simulink model "g"  (Simulink 7.9)
settings: Solver=ode45  StartTime=0.0  StopTime=10.0  RelTol=1e-3
libraries: dspsigops x2
settings Model: Creator=Mihail  LastModifiedBy=Mihail
settings ConfigurationSet: Description=SimMechanics 2G

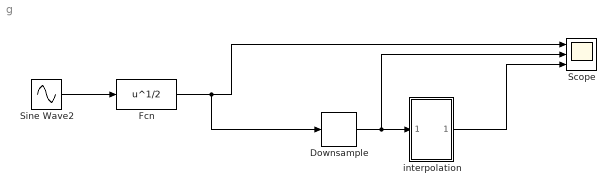
== system g ==
  Downsample : dspsigops/Downsample  N=4  phase=0  RateOptions=Enforce single-rate processing  smode=Allow multirate  fmode=Maintain input frame size  ic=0
  Fcn : Fcn  Expr=u^1/2
  Scope : Scope  NumInputPorts=3
      settings: YMin=-5~-5~-5  YMax=5~5~5
  Sine Wave2 : Sin  Amplitude=1000  Frequency=4  Phase=2*pi  SampleTime=0.01  VectorParams1D=off
  interpolation : Subsystem
  wires:
  Downsample/1 -> interpolation/1(In1), Scope/2
  interpolation/1(Out1) -> Scope/3
  Sine Wave2/1 -> Fcn/1
  Fcn/1 -> Scope/1, Downsample/1

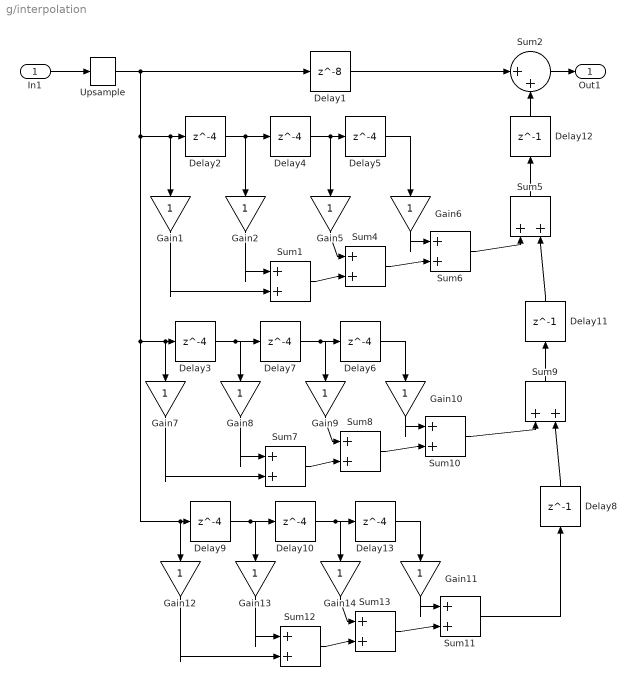
== system g/interpolation ==
  In1 : Inport
  Delay1 : Delay  DelayLength=8
  Delay{2..7,9..10,13} (9 alike) : Delay  DelayLength=4
  Delay11 : Delay  DelayLength=1
  Delay12 : Delay  DelayLength=1
  Delay8 : Delay  DelayLength=1
  Gain{1..2,5..14} (12 alike) : Gain  RndMeth=Convergent
  Sum{1..2,4..13} (12 alike) : Sum  Inputs=|++  SaturateOnIntegerOverflow=on
  Upsample : dspsigops/Upsample  N=4  phase=0  InputProcessing=Columns as channels (frame based)  RateOptions=Enforce single-rate processing  ic=0  mode=Unused parameter value
  Out1 : Outport
  wires:
  In1/1 -> Upsample/1
  Sum2/1 -> Out1/1
  Sum5/1 -> Delay12/1
  Delay12/1 -> Sum2/2
  Delay1/1 -> Sum2/1
  Delay11/1 -> Sum5/2
  Sum9/1 -> Delay11/1
  Sum11/1 -> Delay8/1
  Delay8/1 -> Sum9/2
  Delay13/1 -> Gain11/1
  Gain11/1 -> Sum11/1
  Sum13/1 -> Sum11/2
  Gain14/1 -> Sum13/1
  Sum12/1 -> Sum13/2
  Gain13/1 -> Sum12/1
  Gain12/1 -> Sum12/2
  Delay10/1 -> Gain14/1, Delay13/1
  Delay9/1 -> Gain13/1, Delay10/1
  Delay6/1 -> Gain10/1
  Sum10/1 -> Sum9/1
  Gain10/1 -> Sum10/1
  Sum8/1 -> Sum10/2
  Gain9/1 -> Sum8/1
  Sum7/1 -> Sum8/2
  Gain8/1 -> Sum7/1
  Gain7/1 -> Sum7/2
  Delay7/1 -> Gain9/1, Delay6/1
  Delay3/1 -> Gain8/1, Delay7/1
  Sum6/1 -> Sum5/1
  Gain6/1 -> Sum6/1
  Sum4/1 -> Sum6/2
  Gain5/1 -> Sum4/1
  Sum1/1 -> Sum4/2
  Gain2/1 -> Sum1/1
  Gain1/1 -> Sum1/2
  Delay5/1 -> Gain6/1
  Delay4/1 -> Gain5/1, Delay5/1
  Delay2/1 -> Gain2/1, Delay4/1
  Upsample/1 -> Gain12/1, Delay9/1, Gain7/1, Delay3/1, Gain1/1, Delay2/1, Delay1/1
